simulink library "Window_Control"  (Simulink 8.2)
settings: Solver=ode45  StartTime=0.0  StopTime=10.0  RelTol=1e-3
settings Model: Creator=lena.frank  LastModifiedBy=ralf.dott  CovSaveCumulativeToWorkspaceVar=on

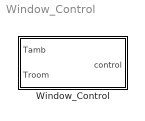
== system Window_Control ==
  Window_Control : Subsystem  mask(Window Control){}
      mask help: Control for free driven passive cooling realized by tilted windows according assuptions of IEA SHC Task44.
      mask Help: web(fullfile(path_carnot('help'),'Window_Control.html'),'-helpbrowser')

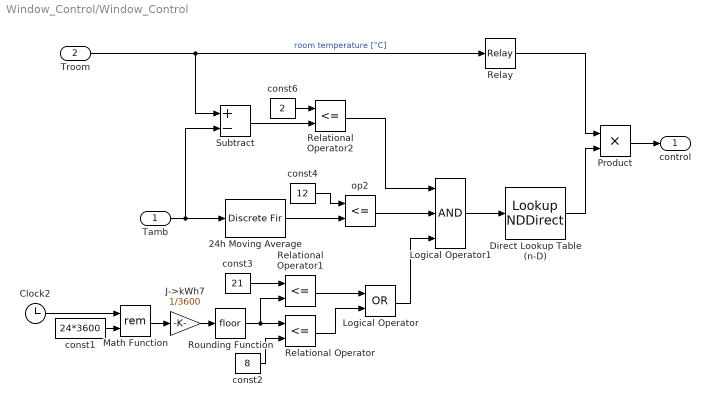
== system Window_Control/Window_Control ==
  Tamb : Inport
  Troom : Inport  Port=2
  24h Moving Average : DiscreteFir  Coefficients=ones(1,24)*(1/24)  SampleTime=3600  AccumDataTypeStr=Inherit: Same as product output  RndMeth=Nearest
  Clock2 : Clock
  Direct Lookup Table (n-D) : LookupNDDirect  NumberOfTableDimensions=1  Table=[0 1]
  J->kWh7 : Gain  Gain=1/3600  SaturateOnIntegerOverflow=on  OutDataTypeStr=Inherit: Same as input  ParamDataTypeStr=Inherit: Same as input
  Logical Operator : Logic  Operator=OR  AllPortsSameDT=off  OutDataTypeStr=boolean
  Logical Operator1 : Logic  Inputs=3  AllPortsSameDT=off  OutDataTypeStr=boolean
  Math Function : Math  Operator=rem  SaturateOnIntegerOverflow=on
  Product : Product  RndMeth=Zero
  Relational Operator : RelationalOperator  Operator=<=  OutDataTypeStr=boolean
  Relational Operator1 : RelationalOperator  Operator=<=  OutDataTypeStr=boolean
  Relational Operator2 : RelationalOperator  Operator=<=  OutDataTypeStr=boolean
  Relay : Relay  OnSwitchValue=24  OffSwitchValue=23
  Rounding Function : Rounding
  Subtract : Sum  Inputs=+-
  const1 : Constant  Value=24*3600
  const2 : Constant  Value=8
  const3 : Constant  Value=21
  const4 : Constant  Value=12
  const6 : Constant  Value=2
  op2 : RelationalOperator  Operator=<=  OutDataTypeStr=boolean
  control : Outport
  wires:
  24h Moving Average/1 -> op2/2
  Relay/1 -> Product/1
  Product/1 -> control/1
  Direct Lookup Table (n-D)/1 -> Product/2
  op2/1 -> Logical Operator1/2
  Logical Operator1/1 -> Direct Lookup Table (n-D)/1
  Relational Operator2/1 -> Logical Operator1/1
  Subtract/1 -> Relational Operator2/2
  const6/1 -> Relational Operator2/1
  Troom/1 -> Subtract/1, Relay/1  "room temperature [°C]"
  Logical Operator/1 -> Logical Operator1/3
  const4/1 -> op2/1
  Tamb/1 -> 24h Moving Average/1, Subtract/2
  Relational Operator/1 -> Logical Operator/2
  Relational Operator1/1 -> Logical Operator/1
  const3/1 -> Relational Operator1/1
  const2/1 -> Relational Operator/2
  Rounding Function/1 -> Relational Operator1/2, Relational Operator/1
  J->kWh7/1 -> Rounding Function/1
  Math Function/1 -> J->kWh7/1
  const1/1 -> Math Function/2
  Clock2/1 -> Math Function/1
